simulink model "Copy_of_calibration_valves"  (R2026a)
settings: Solver=VariableStepAuto  StopTime=inf
StopFcn:
  | az = out.az;
  | 
  | folder = 'calibration_data';
  | 
  | if ~exist(folder, 'dir')
  |     mkdir(folder);
  | end
  | 
  | baseName = 'az_calibration';
  | fileName = fullfile(folder, baseName + ".mat");
  | 
  | n = 2;
  | 
  | while exist(fileName, 'file')
  |     fileName = fullfile(folder, baseName + "_" + n + ".mat");
  |     n = n + 1;
  | end
  | 
  | save(fileName, 'az');
  | 
  | fprintf('Calibration saved to: %s\n', fileName);
values from neighbouring files (symbols this model uses):
  coefficients = [20.111978783 20.2762923351 20.4770477048]    [sensor_calibration.mat]
settings Model: Creator=user  LastModifiedBy=jinyu

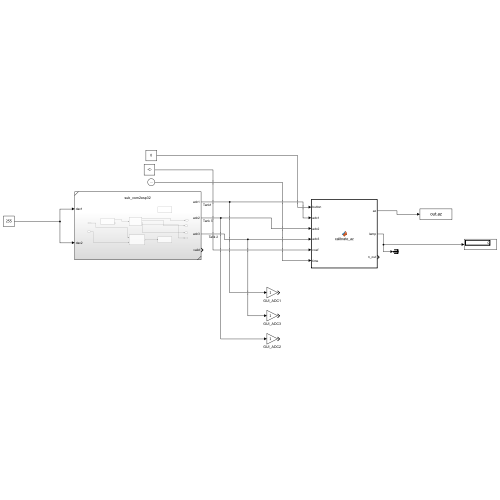
[thumbnail: Simulink's stored preview of the top-level diagram]
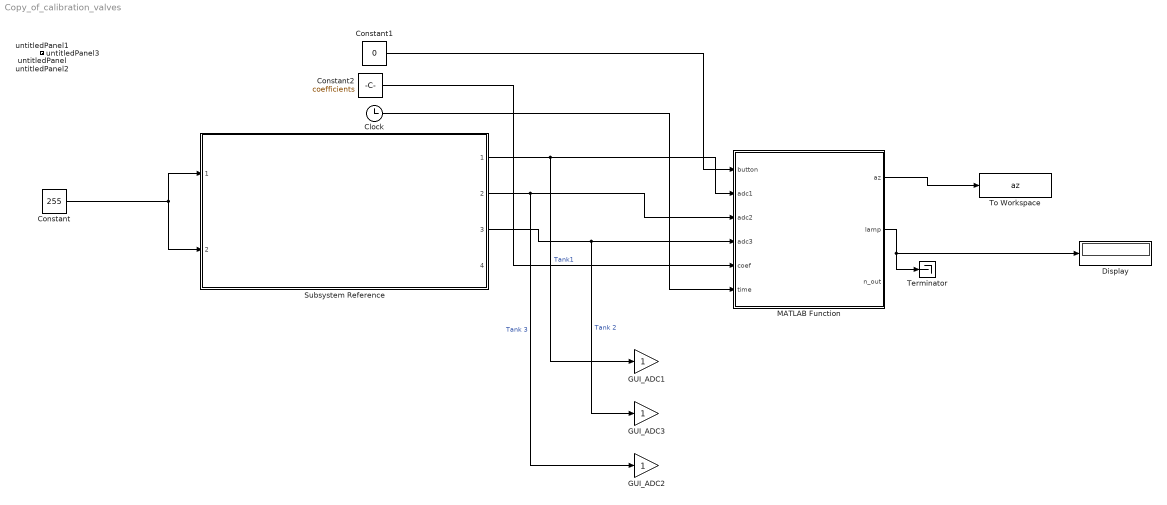
== system Copy_of_calibration_valves ==
  Clock : Clock
  Constant : Constant  Value=255
  Constant1 : Constant  Value=0
  Constant2 : Constant  Value=coefficients
  Display : Display
  GUI_ADC1 : Gain
  GUI_ADC2 : Gain
  GUI_ADC3 : Gain
  MATLAB Function : MATLAB Function  TreatAsAtomicUnit=on
  Subsystem Reference : Subsystem  ReferencedSubsystem=sub_com2esp32
  Terminator : Terminator
  To Workspace : ToWorkspace  VariableName=az  SampleTime=-1
      settings: MaxDataPoints=1
  untitledPanel : Subsystem  Tag=HiddenForWebPanel  IsWebBlockPanel=on
  untitledPanel1 : Subsystem  Tag=HiddenForWebPanel  IsWebBlockPanel=on
  untitledPanel2 : Subsystem  Tag=HiddenForWebPanel  IsWebBlockPanel=on
  untitledPanel3 : Subsystem  Tag=HiddenForWebPanel  IsWebBlockPanel=on
  wires:
  Subsystem Reference/1 -> GUI_ADC1/1, MATLAB Function/2(adc1)  "Tank1"
  MATLAB Function/1(az) -> To Workspace/1
  Constant/1 -> Subsystem Reference/2, Subsystem Reference/1
  Clock/1 -> MATLAB Function/6(time)
  Constant1/1 -> MATLAB Function/1(button)
  Subsystem Reference/2 -> GUI_ADC2/1, MATLAB Function/3(adc2)  "Tank 3"
  Subsystem Reference/3 -> GUI_ADC3/1, MATLAB Function/4(adc3)  "Tank 2"
  MATLAB Function/2(lamp) -> Display/1, Terminator/1
  Constant2/1 -> MATLAB Function/5(coef)

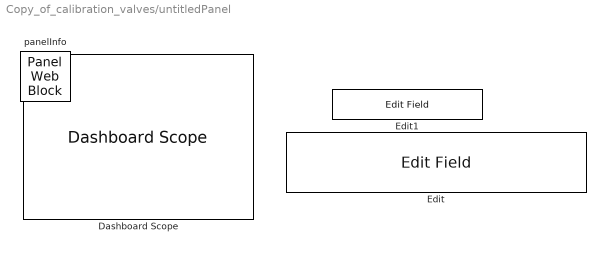
== system Copy_of_calibration_valves/untitledPanel ==
  Dashboard Scope : DashboardScope  Tag=HiddenForWebPanel  PanelInfo="{\"height\":195,\"left\":22,\"panelId\":\"panelId-0a8f6d05-5e0e-4052-8464-4cdde78ccbfe\",\"top\":22,\"type\":\"panelChild\",\"version\":\"2019b\",\"width\":271,\"zIndex\":1500002}"  FontColor=[0.0, 0.0, 0.0]
  Edit : EditField  Tag=HiddenForWebPanel  PanelInfo="{\"height\":25,\"left\":322,\"panelId\":\"panelId-0a8f6d05-5e0e-4052-8464-4cdde78ccbfe\",\"top\":100,\"type\":\"panelChild\",\"version\":\"2019b\",\"width\":181,\"zIndex\":1500006}"  LabelPosition=Hide  ShowInitialText=on  Alignment=Center
  Edit1 : EditField  Tag=HiddenForWebPanel  PanelInfo="{\"height\":30,\"left\":327,\"panelId\":\"panelId-0a8f6d05-5e0e-4052-8464-4cdde78ccbfe\",\"top\":53,\"type\":\"panelChild\",\"version\":\"2019b\",\"width\":150,\"zIndex\":1500004}"  LabelPosition=Hide  ShowInitialText=on  Alignment=Center
  panelInfo : PanelWebBlock  Tag=HiddenForWebPanel  PanelInfo="{\"compacted\":false,\"height\":362,\"isActiveTab\":false,\"left\":183,\"name\":\"Panel\",\"panelId\":\"panelId-0a8f6d05-5e0e-4052-8464-4cdde78ccbfe\",\"popoutData\":{\"height\":495,\"left\":546,\"maximized\":false,\"top\":827,\"width\":618},\"popoutMode\":\"windowHidden\",\"tabIndex\":0,\"tabbedSetId\":\"tabbedSet4972758365\",\"top\":737,\"type\":\"panel\",\"version\":\"2019b\",\"visible\":false,\"width\":602,\"zIndex\":1500002}"  PanelSnapshot=<binary blob, 20028 chars, not shown>

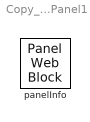
== system Copy_of_calibration_valves/untitledPanel1 ==
  panelInfo : PanelWebBlock  Tag=HiddenForWebPanel  PanelInfo="{\"compacted\":false,\"height\":362,\"isActiveTab\":true,\"left\":183,\"name\":\"Panel1\",\"panelId\":\"panelId-b2ee2f41-7720-49f1-b51a-3062c351f597\",\"popoutData\":{\"height\":495,\"left\":546,\"maximized\":false,\"top\":827,\"width\":618},\"popoutMode\":\"windowHidden\",\"tabIndex\":1,\"tabbedSetId\":\"tabbedSet4972758365\",\"top\":737,\"type\":\"panel\",\"version\":\"2019b\",\"visible\":true,\"width\":602,\"zIndex\":1500004}"

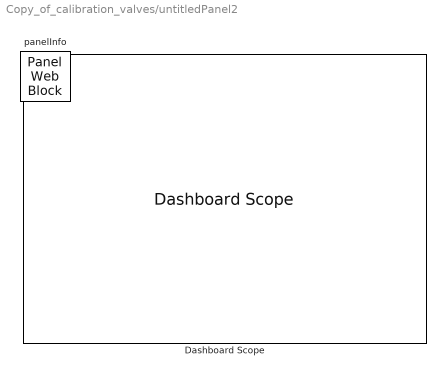
== system Copy_of_calibration_valves/untitledPanel2 ==
  Dashboard Scope : DashboardScope  Tag=HiddenForWebPanel  PanelInfo="{\"height\":289,\"left\":18,\"panelId\":\"panelId-8ba459e9-7eb9-43d1-9a8b-2b7bff5a2d5c\",\"top\":18,\"type\":\"panelChild\",\"version\":\"2019b\",\"width\":403,\"zIndex\":1500002}"  FontColor=[0.0, 0.0, 0.0]
  panelInfo : PanelWebBlock  Tag=HiddenForWebPanel  PanelInfo="{\"compacted\":false,\"height\":329,\"isActiveTab\":true,\"left\":1320,\"name\":\"Panel2\",\"panelId\":\"panelId-8ba459e9-7eb9-43d1-9a8b-2b7bff5a2d5c\",\"popoutData\":{\"height\":440,\"left\":1683,\"maximized\":false,\"top\":822,\"width\":459},\"popoutMode\":\"windowHidden\",\"tabIndex\":0,\"tabbedSetId\":\"tabbedSet1724704130\",\"top\":710,\"type\":\"panel\",\"version\":\"2019b\",\"visible\":true,\"width\":443,\"zIndex\":1500006}"  PanelSnapshot=<binary blob, 75208 chars, not shown>

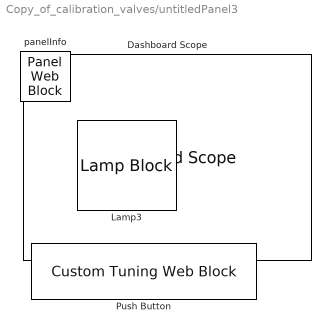
== system Copy_of_calibration_valves/untitledPanel3 ==
  Dashboard Scope : DashboardScope  Tag=HiddenForWebPanel  PanelInfo="{\"height\":461,\"left\":236,\"panelId\":\"panelId-037cc253-1a0e-430c-bfc3-d197bdfa8fb6\",\"top\":13,\"type\":\"panelChild\",\"version\":\"2019b\",\"width\":556,\"zIndex\":1500002}"  FontColor=[0.0, 0.0, 0.0]
  Lamp3 : LampBlock  Tag=HiddenForWebPanel  PanelInfo="{\"height\":68,\"left\":30,\"panelId\":\"panelId-037cc253-1a0e-430c-bfc3-d197bdfa8fb6\",\"top\":30,\"type\":\"panelChild\",\"version\":\"2019b\",\"width\":79,\"zIndex\":1500014}"  LabelPosition=Hide  DefaultColor=[192.0, 192.0, 192.0]
  Push Button : CustomTuningWebBlock  Tag=HiddenForWebPanel  PanelInfo="{\"height\":52,\"left\":27,\"panelId\":\"panelId-037cc253-1a0e-430c-bfc3-d197bdfa8fb6\",\"top\":105,\"type\":\"panelChild\",\"version\":\"2019b\",\"width\":209,\"zIndex\":1500008}"  LabelPosition=Hide  ShowInitialText=on  Configuration="{\"components\":[{\"name\":\"BackgroundImageComponent\",\"settings\":{\"image\":{\"size\":[0,0],\"src\":\"default\",\"srcOrientation\":\"horizontal\"},\"position\":[0,0,1,1],\"scaleMode\":\"0\"}},{\"name\":\"ButtonStateComponent\",\"settings\":{\"buttonType\":\"momentary\",\"clickFcn\":\"\",\"image\":{\"size\":[180,45],\"srcOrientation\":\"Right\"},\"latched\":false,\"offValue\":[],\"onValue\":1,\"position\":[0,0,1,1],\"pressDelay\":500,\"pressFcn\":\"\",\"repeatInterval\":0,\"states\":[{\"horizontalAlignment\":\"center\",\"image\":{\"position\":[0.05,0.015,0.98,0.9],\"size\":[0.98,0.9],\"src\":\"data:image\\/svg+xml;base64,PHN2ZyB4bWxucz0iaHR0cDovL3d3dy53My5vcmcvMjAwMC9zdmciIHhtbG5zOnhsaW5rPSJodHRwOi8vd3d3LnczLm9yZy8xOTk5L3hsaW5rIiB2aWV3Qm94PSIwIDAgMTc3LjI1IDQwLjg4Ij48ZGVmcz48c3R5bGU+LmNscy0xe2ZpbGw6dXJsKCNyYWRpYWwtZ3JhZGllbnQpO30uY2xzLTJ7ZmlsbDp1cmwoI2xpbmVhci1ncmFkaWVudCk7fS5jbHMtM3tmaWxsOnVybCgjbGluZWFyLWdyYWRpZW50LTIpO308L3N0eWxlPjxyYWRpYWxHcmFkaWVudCBpZD0icmFkaWFsLWdyYWRpZW50IiBjeD0iOTAuMDkiIGN5PSIyMi42NiIgcj0i ...(+2212 chars)\",\"srcOrientation\":\"Right\"},\"label\":{\"color\":[1,1,0.78,1],\"icon\":{\"size\":[1.2,1.2],\"src\":\"data:image\\/svg+xml;base64,PHN2ZyBpZD0iT2ZmIiB4bWxucz0iaHR0cDovL3d3dy53My5vcmcvMjAwMC9zdmciIHhtbG5zOnhsaW5rPSJodHRwOi8vd3d3LnczLm9yZy8xOTk5L3hsaW5rIiB2aWV3Qm94PSIwIDAgNTAgNTAiPjxkZWZzPjxzdHlsZT4uY2xzLTF7ZmlsbDojN2Y4MDgwO3N0cm9rZTojMjcyNjI2O3N0cm9rZS1taXRlcmxpbWl0OjEwO3N0cm9rZS13aWR0aDozcHg7fS5jbHMtMntmaWxsOnVybCgjbGluZWFyLWdyYWRpZW50KTt9PC9zdHlsZT48bGluZWFyR3JhZGllbnQgaWQ9ImxpbmVhci1ncmFkaWVudCIgeDE9IjI1IiB5MT0iOSIgeDI9IjI1IiB5Mj0iMzciIGdyYWRpZW50VW5pdHM9InVzZXJTcGFjZU9uVXNlIj48c3RvcCBvZmZzZXQ9IjAiIHN0b3AtY29sb3I9IiNmZmYiIHN0b3Atb3BhY2l0eT0iMC43NSIvPjxzdG9wIG9mZnNldD0iMSIgc3RvcC1jb2xvcj0iI2ZmZiIgc3RvcC1vcGFjaXR5PSIwIi8+PC9saW5lYXJHcmFkaWVudD48L2RlZnM+PGNpcmNsZSBjbGFzcz0iY2xzLTEiIGN4PSIyNSIgY3k9IjI1IiByPSIyMCIvPjxjaXJjbGUgY2xhc3M9ImNscy0yIiBjeD0iMjUiIGN5PSIyMyIgcj0iMTQiLz48L3N2Zz4=\",\"srcOrientation\":\"Right\"},\"iconOffset\":0,\"iconPlacement\":\"left\",\"opacity\":1,\"show\":true,\"text\":{\"content\":\"Button\",\"font\":\"Helvetica\"}},\"labelOffset\":[-0.025,0],\"verticalAlignment\":\"middle\"},{\"horizontalAlignment\":\"center\",\"image\":{\"position\":[0.05,0.015,0.98,0.9],\"size\":[0.98,0.9],\"src\":\"data:image\\/svg+xml;base64,PHN2ZyB4bWxucz0iaHR0cDovL3d3dy53My5vcmcvMjAwMC9zdmciIHhtbG5zOnhsaW5rPSJodHRwOi8vd3d3LnczLm9yZy8xOTk5L3hsaW5rIiB2aWV3Qm94PSIwIDAgMTc3LjI1IDQwLjg4Ij48ZGVmcz48c3R5bGU+LmNscy0xe2ZpbGw6dXJsKCNyYWRpYWwtZ3JhZGllbnQpO30uY2xzLTJ7ZmlsbDp1cmwoI2xpbmVhci1ncmFkaWVudCk7fS5jbHMtM3tmaWxsOnVybCgjbGluZWFyLWdyYWRpZW50LTIpO308L3N0eWxlPjxyYWRpYWxHcmFkaWVudCBpZD0icmFkaWFsLWdyYWRpZW50IiBjeD0iOTAuMDkiIGN5PSIyMi42NiIgcj0i ...(+2216 chars)\",\"srcOrientation\":\"Right\"},\"label\":{\"color\":[1,1,0.78,1],\"icon\":{\"size\":[1.2,1.2],\"src\":\"data:image\\/svg+xml;base64,PHN2ZyB4bWxucz0iaHR0cDovL3d3dy53My5vcmcvMjAwMC9zdmciIHhtbG5zOnhsaW5rPSJodHRwOi8vd3d3LnczLm9yZy8xOTk5L3hsaW5rIiB2aWV3Qm94PSIwIDAgNTAgNTAiPjxkZWZzPjxzdHlsZT4uY2xzLTF7ZmlsbDojNmFiZDQ1O3N0cm9rZTojMjcyNjI2O3N0cm9rZS1taXRlcmxpbWl0OjEwO3N0cm9rZS13aWR0aDozcHg7fS5jbHMtMntmaWxsOnVybCgjbGluZWFyLWdyYWRpZW50KTt9PC9zdHlsZT48bGluZWFyR3JhZGllbnQgaWQ9ImxpbmVhci1ncmFkaWVudCIgeDE9IjI1IiB5MT0iOSIgeDI9IjI1IiB5Mj0iMzciIGdyYWRpZW50VW5pdHM9InVzZXJTcGFjZU9uVXNlIj48c3RvcCBvZmZzZXQ9IjAiIHN0b3AtY29sb3I9IiNmZmYiIHN0b3Atb3BhY2l0eT0iMC43NSIvPjxzdG9wIG9mZnNldD0iMSIgc3RvcC1jb2xvcj0iI2ZmZiIgc3RvcC1vcGFjaXR5PSIwIi8+PC9saW5lYXJHcmFkaWVudD48L2RlZnM+PGcgaWQ9Ik9uIj48Y2lyY2xlIGNsYXNzPSJjbHMtMSIgY3g9IjI1IiBjeT0iMjUiIHI9IjIwIi8+PGNpcmNsZSBjbGFzcz0iY2xzLTIiIGN4PSIyNSIgY3k9IjIzIiByPSIxNCIvPjwvZz48L3N2Zz4=\",\"srcOrientation\":\"Right\"},\"iconOffset\":0,\"iconPlacement\":\"left\",\"opacity\":1,\"show\":true,\"text\":{\"content\":\"Button\",\"font\":\"Helvetica\"}},\"labelOffset\":[0,0],\"verticalAlignment\":\"middle\"},{\"horizontalAlignment\":\"center\",\"image\":{\"position\":[0.05,0.015,0.98,0.9],\"size\":[0.98,0.9],\"src\":\"data:image\\/svg+xml;base64,PHN2ZyB4bWxucz0iaHR0cDovL3d3dy53My5vcmcvMjAwMC9zdmciIHhtbG5zOnhsaW5rPSJodHRwOi8vd3d3LnczLm9yZy8xOTk5L3hsaW5rIiB2aWV3Qm94PSIwIDAgMTc3LjI1IDQwLjg4Ij48ZGVmcz48c3R5bGU+LmNscy0xe2ZpbGw6dXJsKCNyYWRpYWwtZ3JhZGllbnQpO30uY2xzLTJ7ZmlsbDp1cmwoI2xpbmVhci1ncmFkaWVudCk7fS5jbHMtM3tmaWxsOnVybCgjbGluZWFyLWdyYWRpZW50LTIpO308L3N0eWxlPjxyYWRpYWxHcmFkaWVudCBpZD0icmFkaWFsLWdyYWRpZW50IiBjeD0iOTAuMDkiIGN5PSIyMi42NiIgcj0i ...(+2212 chars)\",\"srcOrientation\":\"Right\"},\"label\":{\"color\":[1,1,0.78,1],\"icon\":{\"size\":[1.2,1.2],\"src\":\"data:image\\/svg+xml;base64,PHN2ZyB4bWxucz0iaHR0cDovL3d3dy53My5vcmcvMjAwMC9zdmciIHhtbG5zOnhsaW5rPSJodHRwOi8vd3d3LnczLm9yZy8xOTk5L3hsaW5rIiB2aWV3Qm94PSIwIDAgNTAgNTAiPjxkZWZzPjxzdHlsZT4uY2xzLTF7ZmlsbDojNmFiZDQ1O3N0cm9rZTojMjcyNjI2O3N0cm9rZS1taXRlcmxpbWl0OjEwO3N0cm9rZS13aWR0aDozcHg7fS5jbHMtMntmaWxsOnVybCgjbGluZWFyLWdyYWRpZW50KTt9PC9zdHlsZT48bGluZWFyR3JhZGllbnQgaWQ9ImxpbmVhci1ncmFkaWVudCIgeDE9IjI1IiB5MT0iOSIgeDI9IjI1IiB5Mj0iMzciIGdyYWRpZW50VW5pdHM9InVzZXJTcGFjZU9uVXNlIj48c3RvcCBvZmZzZXQ9IjAiIHN0b3AtY29sb3I9IiNmZmYiIHN0b3Atb3BhY2l0eT0iMC43NSIvPjxzdG9wIG9mZnNldD0iMSIgc3RvcC1jb2xvcj0iI2ZmZiIgc3RvcC1vcGFjaXR5PSIwIi8+PC9saW5lYXJHcmFkaWVudD48L2RlZnM+PGcgaWQ9Ik9uIj48Y2lyY2xlIGNsYXNzPSJjbHMtMSIgY3g9IjI1IiBjeT0iMjUiIHI9IjIwIi8+PGNpcmNsZSBjbGFzcz0iY2xzLTIiIGN4PSIyNSIgY3k9IjIzIiByPSIxNCIvPjwvZz48L3N2Zz4=\",\"srcOrientation\":\"Right\"},\"iconOffset\":0,\"iconPlacement\":\"left\",\"opacity\":1,\"show\":true,\"text\":{\"content\":\"Button\",\"font\":\"Helvetica\"}},\"labelOffset\":[-0.025,0],\"verticalAlignment\":\"middle\"},{\"horizontalAlignment\":\"center\",\"image\":{\"position\":[0.05,0.015,0.98,0.9],\"size\":[0.98,0.9],\"src\":\"data:image\\/svg+xml;base64,PHN2ZyB4bWxucz0iaHR0cDovL3d3dy53My5vcmcvMjAwMC9zdmciIHhtbG5zOnhsaW5rPSJodHRwOi8vd3d3LnczLm9yZy8xOTk5L3hsaW5rIiB2aWV3Qm94PSIwIDAgMTc3LjI1IDQwLjg4Ij48ZGVmcz48c3R5bGU+LmNscy0xe2ZpbGw6dXJsKCNyYWRpYWwtZ3JhZGllbnQpO30uY2xzLTJ7ZmlsbDp1cmwoI2xpbmVhci1ncmFkaWVudCk7fS5jbHMtM3tmaWxsOnVybCgjbGluZWFyLWdyYWRpZW50LTIpO308L3N0eWxlPjxyYWRpYWxHcmFkaWVudCBpZD0icmFkaWFsLWdyYWRpZW50IiBjeD0iOTAuMDkiIGN5PSIyMi42NiIgcj0i ...(+2216 chars)\",\"srcOrientation\":\"Right\"},\"label\":{\"color\":[1,1,0.78,1],\"icon\":{\"size\":[1.2,1.2],\"src\":\"data:image\\/svg+xml;base64,PHN2ZyBpZD0iT2ZmIiB4bWxucz0iaHR0cDovL3d3dy53My5vcmcvMjAwMC9zdmciIHhtbG5zOnhsaW5rPSJodHRwOi8vd3d3LnczLm9yZy8xOTk5L3hsaW5rIiB2aWV3Qm94PSIwIDAgNTAgNTAiPjxkZWZzPjxzdHlsZT4uY2xzLTF7ZmlsbDojN2Y4MDgwO3N0cm9rZTojMjcyNjI2O3N0cm9rZS1taXRlcmxpbWl0OjEwO3N0cm9rZS13aWR0aDozcHg7fS5jbHMtMntmaWxsOnVybCgjbGluZWFyLWdyYWRpZW50KTt9PC9zdHlsZT48bGluZWFyR3JhZGllbnQgaWQ9ImxpbmVhci1ncmFkaWVudCIgeDE9IjI1IiB5MT0iOSIgeDI9IjI1IiB5Mj0iMzciIGdyYWRpZW50VW5pdHM9InVzZXJTcGFjZU9uVXNlIj48c3RvcCBvZmZzZXQ9IjAiIHN0b3AtY29sb3I9IiNmZmYiIHN0b3Atb3BhY2l0eT0iMC43NSIvPjxzdG9wIG9mZnNldD0iMSIgc3RvcC1jb2xvcj0iI2ZmZiIgc3RvcC1vcGFjaXR5PSIwIi8+PC9saW5lYXJHcmFkaWVudD48L2RlZnM+PGNpcmNsZSBjbGFzcz0iY2xzLTEiIGN4PSIyNSIgY3k9IjI1IiByPSIyMCIvPjxjaXJjbGUgY2xhc3M9ImNscy0yIiBjeD0iMjUiIGN5PSIyMyIgcj0iMTQiLz48L3N2Zz4=\",\"srcOrientation\":\"Right\"},\"iconOffset\":0,\"iconPlacement\":\"left\",\"opacity\":1,\"show\":true,\"text\":{\"content\":\"Button\",\"font\":\"Helvetica\"}},\"labelOffset\":[0,0],\"verticalAlignment\":\"middle\"}]}},{\"name\":\"ForegroundImageComponent\",\"settings\":{\"image\":{\"size\":[0,0],\"src\":\"default\",\"srcOrientation\":\"horizontal\"},\"isForeground\":1,\"position\":[0,0,1,1],\"scaleMode\":\"0\"}}],\"derived\":{\"blockParameters\":{\"AutoActivate\":false,\"ButtonText\":\"Button\",\"ButtonType\":\"Momentary\",\"ClickFcn\":\"\",\"OnValue\":1,\"PressDelay\":500,\"PressFcn\":\"\",\"RepeatInterval\":0,\"fixedAspectRatio\":\"on\"}},\"settings\":{\"BindingType\":\"param\",\"aspectRatio\":3.7777777777777777,\"autoActivate\":false,\"backgroundColor\":[0,0,0,\"1\"],\"backgroundOffset\":0,\"backgroundOpacity\":1,\"fixedAspectRatio\":\"on\",\"foregroundColor\":[252,252,196],\"showBackgroundColor\":false,\"variant\":\"push\",\"version\":\"R2025a\"},\"type\":\"Button\"}"
  panelInfo : PanelWebBlock  Tag=HiddenForWebPanel  PanelInfo="{\"compacted\":false,\"height\":495,\"isActiveTab\":true,\"labels\":{},\"left\":1232,\"name\":\"Panel3\",\"panelId\":\"panelId-037cc253-1a0e-430c-bfc3-d197bdfa8fb6\",\"tabIndex\":0,\"tabbedSetId\":\"tabbedSet3591606152\",\"top\":300,\"type\":\"panel\",\"version\":\"2019b\",\"visible\":true,\"width\":798,\"zIndex\":1500008}"  PanelSnapshot=<binary blob, 36164 chars, not shown>

== matlab function Copy_of_calibration_valves/MATLAB Function ==
  data: button input; adc1 input; adc2 input; adc3 input; coef input; az output; lamp output; time input; n_out output
function [az, lamp, n_out] = calibrate_az(button, adc1, adc2, adc3, coef, time)

persistent running t_start ...
           h1_start h2_start h3_start ...
           az_out

lamp  = 0;
n_out = 0;

if isempty(running)
    running  = 0;
    t_start  = 0;

    h1_start = 0;
    h2_start = 0;
    h3_start = 0;

    az_out   = zeros(3,1);
end

A  = 154.0;
Sn = 0.5;
g  = 981.0;


x1 = adc1(1);
x2 = adc3(1);
x3 = adc2(1);

h1 = ((coef(1,1) * x1 + coef(1,2)) * x1 ...
      + coef(1,3)) * x1 + coef(1,4);

h2 = ((coef(2,1) * x2 + coef(2,2)) * x2 ...
      + coef(2,3)) * x2 + coef(2,4);

h3 = ((coef(3,1) * x3 + coef(3,2)) * x3 ...
      + coef(3,3)) * x3 + coef(3,4);

t = time(1);
b = button(1);

if b > 0.5 && running == 0 && ...
        h1 > 5 && h2 > 5 && h3 > 5

    running  = 1;
    t_start  = t;

    h1_start = h1;
    h2_start = h2;
    h3_start = h3;

    az_out   = zeros(3,1);
end

if running == 1

    lamp  = 1;
    n_out = t - t_start;

    if (t - t_start) >= 60

        dt = t - t_start;

        h1_end = h1;
        h2_end = h2;
        h3_end = h3;

        dh1 = h1_start - h1_end;
        dh2 = h2_start - h2_end;
        dh3 = h3_start - h3_end;

        h1m = (h1_start + h1_end) / 2;
        h2m = (h2_start + h2_end) / 2;
        h3m = (h3_start + h3_end) / 2;

        d13 = max(h1m - h3m, 1e-6);
        d32 = max(h3m - h2m, 1e-6);
        h20 = max(h2m, 1e-6);

        az1 = A * dh1 / ...
            (dt * Sn * sqrt(2 * g * d13));

        az2 = A * (dh1 + dh2 + dh3) / ...
            (dt * Sn * sqrt(2 * g * h20));

        az3 = A * (dh1 + dh3) / ...
            (dt * Sn * sqrt(2 * g * d32));

        az_out = [az1; az2; az3];

        running = 2;
    end
end

if running == 2
    lamp  = 2;
    n_out = 60;
end

az = az_out;
end
